simulink model "dspvorbisdec"  (Simulink 8.3)
settings: Solver=FixedStepDiscrete  SolverMode=SingleTasking  StartTime=0.0  StopTime=inf  RelTol=1e-3
PostLoadFcn:
  | hws  = get_param(bdroot,'modelworkspace');
  | dspvorbisdec_SampRt = hws.evalin('dspvorbisdec_OutputSampRt');
  | clear hws;
StopFcn:
  | dspvorbisdec_hws = get_param(bdroot,'modelworkspace');
  | dspvorbisdec_tmp = dspvorbisdec_hws.data;
  | for i = 1:length(dspvorbisdec_tmp)
  |   if strcmp(dspvorbisdec_tmp(i).Name,'dspvorbisdec_OutputSampRt')
  |      if (dspvorbisdec_tmp(i).Value~=dspvorbisdec_SampRt)
  |         dspvorbisdec_hws.assignin('dspvorbisdec_OutputSampRt', dspvorbisdec_SampRt);
  |      end
  |   end
  | end
  | 
  | clear hws dspvorbisdec_tmp i dspvorbisdec_hws;
undefined symbols (not defined in the file or in its folder): blockSize, errordlg, uiwait, warndlg
libraries: simulink x5, dspmtrx3 x3, dspindex x2, dspsigops x1, dspxfrm3 x1, dspmisc x1, dspsnks4 x1, dspsrcs4 x1
(part 2 of 3)

== matlab function Decode All Pages of Data/decodePage/Decode Audio/Decode an Audio Block/Decode Floor and Residue (4.3.2-4.3.5) ==
  data: resiOut output double; floor1Out output double; ifOutput output double; blockSize input uint32; startBitPoint input double; mapNum input double; dat input double; mapData input double; codeBooks input double; resiData input double; resiDataLocs input double; floor1Data input double; floor1DataLocs input double; numChannels input double; totalBytes input double
function [resiOut, floor1Out, ifOutput] = decodeFloorResidue(blockSize, startBitPoint, mapNum, dat, mapData, codeBooks, resiData, resiDataLocs, floor1Data, floor1DataLocs, numChannels, totalBytes)

persistent floor1_step2_flag1;
if isempty(floor1_step2_flag1)
    floor1_step2_flag1 = uint8(zeros(256,1));
end
persistent floor1_final_Y1;
if isempty(floor1_final_Y1)
    floor1_final_Y1 = uint32(zeros(256,1));
end
persistent floor1_step2_flag;
if isempty(floor1_step2_flag)
    floor1_step2_flag = uint8(zeros(256,1));
end
persistent floor1_final_Y;
if isempty(floor1_final_Y)
    floor1_final_Y = uint32(zeros(256,1));    
end
persistent classifications;
if isempty(classifications)
    classifications = uint32(zeros(256,2)); 
end
persistent uzeros8192;
if isempty (uzeros8192)
    uzeros8192 = uint8(zeros(8192,2));
end
persistent zeros8192;
if isempty(zeros8192)
    zeros8192 = double(zeros(8192,2));
end
persistent zeros256;
if isempty(zeros256)
    zeros256 = uint8(zeros(256,1));
end

persistent data;
if isempty(data)
    data = logical(false(16384, 1));
end
for m = uint32(0):uint32(totalBytes-1)
    for i = eml.unroll(uint32(1):uint32(8))
        data(8*m+i) = bitget(dat(m+1), i); % convert bytestream into bitstream
    end
end


%%%%%%%%%%%%%%%%%%%%%%%%%%%%%%%%%%%%%%%%%%%%%%%%%%%%%%%%%%%%%%%%%%%%%%%%
%%%%%%%%%%%% Decode Floor1 %%%%%%%%%%%%%%%%%%%%%%%%%%%%%%%%%%%%%%%%%%%%%
%%%%%%%%%%%%%%%%%%%%%%%%%%%%%%%%%%%%%%%%%%%%%%%%%%%%%%%%%%%%%%%%%%%%%%%%
% Decoding routines below follow Part 7.2.2 of Vorbis Decoder Specification, most names of variables and parameters are unchanged for better readibility 

bitPoint = startBitPoint;
floor1Out = uzeros8192; % enforce memcpy at code generation
resiOut = zeros8192; % enforce memcpy at code generation

no_residue = uint8(zeros(2,1));
curFloorLen = blockSize/2;

mapNum = mapNum*2;

%Iterate over each channel of 2 channels
for i_ch = 1:numChannels
    bytePoint = uint32(1);
    
    % Check if [no_residue] is set
    bitPoint = bitPoint + uint32(1);
    if ~data(bitPoint-1)
        no_residue(i_ch) = 1;
        continue;
    end
    
    submap_number = mapData(1+mapNum+2, i_ch);
    floor_number = mapData(1+mapNum+2, numChannels+submap_number*2+1)+1;
    
    a = uint32([256, 128, 86, 64]);
    range1 = a(floor1Data(floor1DataLocs(4,floor_number)));

    % ilog() function from the original C-library
    ret = uint32(0);
    v = uint32(range1-1);
    while (v)
        ret = ret+1;
        v = bitshift(v,-1);
    end
    % end of ilog()
    count = ret;

    floor1_Y = zeros256;
    for j = eml.unroll(uint32(1):uint32(2))
        for i = uint32(1):count
            floor1_Y(bytePoint) = bitset(floor1_Y(bytePoint), i, data(bitPoint)); 
            bitPoint = bitPoint + 1;
        end
        bytePoint = bytePoint + 1;
    end

    offset = uint32(2);
    for iter = 0:floor1Data(floor1DataLocs(1,floor_number))-1
        class1 = floor1Data(floor1DataLocs(2,floor_number)+iter);
        ix1 = class1+1+(floor_number-1)*16;
        cdim =  floor1Data(floor1DataLocs(3,ix1));
        cbits = floor1Data(floor1DataLocs(3,ix1)+1);
        csub = bitshift(uint32(1),cbits)-1;
        cval = uint32(0);
        if (cbits)
            book = floor1Data(floor1DataLocs(3,ix1)+2)+1;
            %HUFFMAN DECODE
            huff_bit_count = uint32(0);
            huff_buf = uint32(0);
            ifdecoded = false;
            while (~ifdecoded)
                huff_bit_count = huff_bit_count + 1;
                huff_buf = bitset(huff_buf, huff_bit_count, data(bitPoint));
                for iter_h = codeBooks(2*book-1, 256*30-32+huff_bit_count-1):(codeBooks(2*book-1, 256*30-32+huff_bit_count)-1)
                    if (huff_buf==bitand(codeBooks(2*book, iter_h), bitshift(uint32(1), huff_bit_count)-1))
                        if huff_bit_count == codeBooks(2*book-1, 2+iter_h)
                            cval = codeBooks(2*book, iter_h+codeBooks(2*book-1, 2))-1;
                            ifdecoded = true;
                        end
                        break;
                    end
                end
                bitPoint = bitPoint + 1;
            end
            %END HUFFMAN DECODE                
        end

        for iter_j = 0:cdim-1
            if (cbits)
                book = floor1Data(floor1DataLocs(3,ix1)+3+bitand(cval, csub))+1;
            else
                book = floor1Data(floor1DataLocs(3,ix1)+2+bitand(cval, csub))+1;
            end
            cval = uint32(bitshift(cval, -int32(cbits)));                                                    
            if (book~=256)
                %HUFFMAN DECODE
                huff_bit_count = uint32(0);
                huff_buf = uint32(0);
                ifdecoded = false;
                while (~ifdecoded)
                    huff_bit_count = huff_bit_count + 1;
                    huff_buf = bitset(huff_buf, huff_bit_count, data(bitPoint));
                    for iter_h = codeBooks(2*book-1, 256*30-32+huff_bit_count-1):(codeBooks(2*book-1, 256*30-32+huff_bit_count)-1)
                        if (huff_buf==bitand(codeBooks(2*book, iter_h), bitshift(uint32(1), huff_bit_count)-1))
                            if huff_bit_count == codeBooks(2*book-1, 2+iter_h)
                                floor1_Y(iter_j+offset+1) = codeBooks(2*book, iter_h+codeBooks(2*book-1, 2))-1;
                                ifdecoded = true;
                            end
                            break;                            
                        end
                    end
                    bitPoint = bitPoint + 1;
                end
                %END HUFFMAN DECODE                
            else
                floor1_Y(iter_j+offset+1) = 0;
            end
        end
        offset = offset + cdim;
    end

    % CURVE COMPUTATION
    floor1_step2_flag(1) = 1;
    floor1_step2_flag(2) = 1;                                
    floor1_final_Y(1) = floor1_Y(1);
    floor1_final_Y(2) = floor1_Y(2);
    
    flIx = floor1DataLocs(5, floor_number); % remember this index for further multiple use

    for m = uint32(2):floor1Data(floor1DataLocs(1, floor_number)-1)-1
        % low_neighbor, hi_neigbor
        low_neighbor_offset = uint32(0);
        hi_neighbor_offset = uint32(1);
        lx = int32(0); 
        hx = int32(curFloorLen);
        for q = uint32(0):(m-1)
            if (floor1Data(flIx+q)<floor1Data(flIx+m))
                if (floor1Data(flIx+q)>lx)
                    low_neighbor_offset = q; lx=int32(floor1Data(flIx+q));
                end
            end
            if (floor1Data(flIx+q)>floor1Data(flIx+m))
                if (floor1Data(flIx+q)<hx)
                    hi_neighbor_offset = q; hx=int32(floor1Data(flIx+q));
                end
            end
        end
        %%%%%%%%%%%%%% end %%%%%%%%%%%%%%%%%%

        x0 = int32(floor1Data(flIx+low_neighbor_offset));
        y0 = int32(floor1_final_Y(low_neighbor_offset+1));
        x1 = int32(floor1Data(flIx+hi_neighbor_offset));
        y1 = int32(floor1_final_Y(hi_neighbor_offset+1));
        X = int32(floor1Data(flIx+m));

        % render_point(x0, y0, x1, y1, X)
        dy = y1-y0;
        adx = x1-x0;
        ady = abs(dy);
        err = ady*(X-x0);
        if (adx==0); adx=int32(1); end
        off = (err-rem(err,adx))/adx;
        if (dy<0)
            predicted = y0 - off;
        else
            predicted = y0 + off;
        end
        %%%%%%% end %%%%%%%%%%%%%%

        val = int32(floor1_Y(m+1)); 
        highroom = int32(range1)-predicted;
        lowroom = predicted;
        if (highroom<lowroom)
            room = highroom*2;
        else
            room = lowroom*2;
        end
        if (val)
            floor1_step2_flag(low_neighbor_offset+1) = 1;
            floor1_step2_flag(hi_neighbor_offset+1) = 1;                                        
            floor1_step2_flag(m+1) = 1;
            if val>=room
                if highroom>lowroom
                    floor1_final_Y(m+1) = val-lowroom+predicted;
                else
                    floor1_final_Y(m+1) = predicted-val+highroom-1;
                end
            else
                if (mod(val, 2))
                    floor1_final_Y(m+1) = predicted-(val+1)/2;
                else
                    floor1_final_Y(m+1) = predicted+val/2;
                end
            end
        else
            floor1_step2_flag(m+1) = 0;
            floor1_final_Y(m+1) = predicted;
        end
    end

    n = floor1Data(floor1DataLocs(1, floor_number)-1);
    c = 333333*ones(256, 1);
    for m = flIx:(flIx+n-1)
        c(m-flIx+1) = floor1Data(m);
    end
    [floor1_X_list1, ix] = sort(c);
    for m = 1:n
        floor1_final_Y1(m) = floor1_final_Y(ix(m));
        floor1_step2_flag1(m) = floor1_step2_flag(ix(m));        
    end

    hx = int32(0);
    lx = int32(0);
    hy = int32(0);
    floor1_multiplier = floor1Data(floor1DataLocs(4,floor_number));
    ly = int32(floor1_final_Y1(1)*floor1_multiplier);
    for m = 1:(floor1Data(floor1DataLocs(1, floor_number)-1)-1)
        if (floor1_step2_flag1(m+1))
            hy = int32(floor1_final_Y1(m+1)*floor1_multiplier);
            hx = int32(floor1_X_list1(m+1));

            % Floor rendering routines
            dy = hy - ly;
            adx = hx-lx;
            ady = abs(dy);
            if (adx==0); adx=int32(1); end
            base = (dy-rem(dy,adx))/adx;
            x = lx;
            y = ly;
            err = int32(0);
            if (dy<0); sy = base - 1;
            else sy = base + 1; end
            ady = ady - abs(base)*adx;
            floor1Out(x+1,i_ch) = y;
            
            for x = lx+2:hx
                err = err + ady;
                if (err>=adx)
                    err = err - adx;
                    y = y + sy;
                else
                    y = y + base;
                end

                floor1Out(x,i_ch) = y;
            end            
            % end of line rendering
            lx = hx;
            ly = hy;
        end
    end

    if (hx<=int32(curFloorLen))
        % line rendering routines again
        dy = int32(0);
        adx = int32(curFloorLen) - hx;
        ady = abs(dy);
        if (adx==0); adx=int32(1); end
        base = (dy-rem(dy,adx))/adx;
        x = hx;
        y = hy;
        err = int32(0);
        if (dy<0)
            sy = base - 1;
        else
            sy = base + 1;
        end
        ady = ady - abs(base)*adx;
        floor1Out(x+1,i_ch) = y;
        for x = hx+2:int32(curFloorLen)
            err = err + ady;
            if (err>=adx)
                err = err - adx;
                y = y + sy;
            else
                y = y + base;
            end
            floor1Out(x,i_ch) = y;
        end
        % end of line rendering
    end

end

%%%%%%%%%%%%%%%%%%%%%%%%%%%%%%%%%%%%%%%%%%%%%%%%%%%%%%%%%%%%%%%%%%%%%%%%
%%%%%%%%%%%%%%%%%%%%% Decode residue %%%%%%%%%%%%%%%%%%%%%%%%%%%%%%%%%%%
%%%%%%%%%%%%%%%%%%%%%%%%%%%%%%%%%%%%%%%%%%%%%%%%%%%%%%%%%%%%%%%%%%%%%%%%
% Decoding routines below follow Part 8.6.2 of Vorbis Decoder Specification, most names of variables and parameters are unchanged for better readibility 

if (sum(no_residue)*(numChannels==1)+(sum(no_residue)-1)*(numChannels==2))>0
    ifOutput = 0; % no audio energy in the frame
else
    ifOutput = 1;
end

% 4.3.3 of Vorbis Decoder Specification, nonzero vector propagate
if (mapData(1+mapNum+1,2)>0) % To Avoid overflow error
    for i_sub = 0:mapData(1+mapNum+1,2)-1
        if (~no_residue(mapData(1+mapNum+1,3+i_sub*2)+1))||(~no_residue(mapData(1+mapNum+1,3+i_sub*2+1)+1))
            no_residue(mapData(1+mapNum+1,3+i_sub*2)+1) = 0;
            no_residue(mapData(1+mapNum+1,3+i_sub*2+1)+1) = 0;
        end
    end
end

vorbis_mapping_submaps = mapData(1+mapNum+1,1);
for i_sub = 1:vorbis_mapping_submaps % Iterate vorbis_mapping_submaps times
    do_not_decode_flag = uint8(zeros(2,1));
    ch_tmp = uint32(0);
    for j_ch = uint32(0):numChannels-1
        if (mapData(1+mapNum+2,j_ch+1)==i_sub-1)
            if (no_residue(j_ch+1))
                do_not_decode_flag(ch_tmp+1) = 1;
            end
            ch_tmp = ch_tmp + 1;
        end
    end

    resi_number = mapData(1+mapNum+2,numChannels+i_sub*2)+1; 
    resi_type = resiData(resiDataLocs(1,resi_number)-2);

    ch = ch_tmp;
    if (resi_type == 2)
        ch = uint32(1);
    end
    
    book = resiData(resiDataLocs(1,resi_number)+10)+1;
    classwords_per_codeword = int32(codeBooks(2*book-1, 1));

    residue_begin = resiData(resiDataLocs(1,resi_number))+bitshift(uint32(resiData(resiDataLocs(1,resi_number)+1)), 8)+bitshift(uint32(resiData(resiDataLocs(1,resi_number)+2)), 16);
    residue_end = resiData(resiDataLocs(1,resi_number)+3)+bitshift(uint32(resiData(resiDataLocs(1,resi_number)+4)), 8)+bitshift(uint32(resiData(resiDataLocs(1,resi_number)+5)), 16);
    residue_partition_size = resiData(resiDataLocs(1,resi_number)+6)+bitshift(uint32(resiData(resiDataLocs(1,resi_number)+7)), 8)+bitshift(uint32(resiData(resiDataLocs(1,resi_number)+8)), 16) + 1;
    n_to_read = residue_end - residue_begin;
    partitions_to_read = n_to_read/residue_partition_size;

    iter_step = 1;
    for iter_pass = uint32(0):resiData(resiDataLocs(1,resi_number)-1)-1 %look->stages loop
        partition_count = 0;
        while partition_count<partitions_to_read % partvals loop
            if (iter_pass==0)
                for j_ch = uint32(1):ch
                    if (do_not_decode_flag(j_ch)); continue; end;
                    
                    %HUFFMAN DECODE
                    huff_bit_count = uint32(0);
                    huff_buf = uint32(0);
                    temp = uint32(0);
                    ifdecoded = false;
                    while (~ifdecoded)
                        huff_bit_count = huff_bit_count + 1;
                        huff_buf = bitset(huff_buf, huff_bit_count, data(bitPoint));
                        for iter_h = codeBooks(2*book-1, 256*30-32+huff_bit_count-1):(codeBooks(2*book-1, 256*30-32+huff_bit_count)-1)
                            if (huff_buf==bitand(codeBooks(2*book, iter_h), bitshift(uint32(1), huff_bit_count)-1))
                                if huff_bit_count == codeBooks(2*book-1, 2+iter_h)
                                    temp = codeBooks(2*book, iter_h+codeBooks(2*book-1, 2))-1;
                                    ifdecoded = true;
                                end
                                break;
                            end
                        end
                        bitPoint = bitPoint + 1;
                    end
                    %END HUFFMAN DECODE                    
                    for k = (classwords_per_codeword-1):-1:0
                        classifications(k+partition_count+1,j_ch) = mod(temp, resiData(resiDataLocs(1,resi_number)+9)); % Modified for stereo
                        temp = (temp-classifications(k+partition_count+1,j_ch))/resiData(resiDataLocs(1,resi_number)+9);
                    end
                end
            end


            for iter_i = 0:(classwords_per_codeword-1)
                if (partition_count<partitions_to_read)
                    for j_ch = 1:ch
                        if (do_not_decode_flag(j_ch));
                            partition_count = partition_count + 1;                            
                            continue; 
                        end;                        
                        vqclass1 = classifications(partition_count+1,j_ch);% Modified for stereo
                        vqbook = resiData(resiDataLocs(2, resi_number)+vqclass1*8 + iter_pass) + 1;
                        vqIx = vqbook*2;
                        if (vqbook~=256)

                            offset = residue_begin+partition_count*residue_partition_size;
                            step = uint32(0);
                            switch resi_type
                                case 0
                                    step = (residue_partition_size-rem(residue_partition_size,codeBooks(vqIx-1, 1)))/codeBooks(vqIx-1, 1);
                                case {1, 2}
                                    step = residue_partition_size;
                            end

                            while (iter_step<=step)

                                %HUFFMAN DECODE
                                huff_bit_count = uint32(0);
                                huff_buf = uint32(0);
                                lookup_offset = uint32(0);
                                ifdecoded = false;
                                while (~ifdecoded)
                                    huff_bit_count = huff_bit_count + 1;
                                    huff_buf = uint32(bitset(huff_buf, huff_bit_count, data(bitPoint)));
                                    for iter_h = codeBooks(vqIx-1, 256*30-32+huff_bit_count-1):(codeBooks(vqIx-1, 256*30-32+huff_bit_count)-1)
                                        if (huff_buf==bitand(codeBooks(vqIx, iter_h), bitshift(uint32(1), huff_bit_count)-1))
                                            if huff_bit_count == codeBooks(vqIx-1, 2+iter_h)
                                                lookup_offset = codeBooks(vqIx, iter_h+codeBooks(vqIx-1, 2))-1;
                                                ifdecoded = true;
                                            end
                                            break;
                                        end
                                    end
                                    bitPoint = bitPoint + 1;
                                end
                                %END HUFFMAN DECODE                    


                                xr = codeBooks(vqIx-1, 3+codeBooks(vqIx-1, 2)+1);
                                mantissa = double(bitand(xr, 2097151));
                                sign1 = bitand(xr, 2147483648);
                                exponent = double(bitshift(uint32(bitand(xr, 2145386496)), -21));
                                if sign1; mantissa=-mantissa; end
                                codebook_minimum_value = int32(mantissa*(2^(exponent-788)));                        

                                xr = codeBooks(vqIx-1, 3+codeBooks(vqIx-1, 2)+2);
                                mantissa = double(bitand(xr, 2097151));
                                sign1 = bitand(xr, 2147483648);
                                exponent = double(bitshift(uint32(bitand(xr, 2145386496)), -21));
                                if sign1; mantissa=-mantissa; end
                                codebook_delta_value = int32(mantissa*(2^(exponent-788))); 
                                value_vector = int32(zeros(32,2)); 

                                if (codeBooks(vqIx-1, 3+codeBooks(vqIx-1, 2))==1)
                                    last = int32(0);
                                    index_divisor = uint32(1);
                                    for iter_h = 0:(codeBooks(vqIx-1, 1)-1)
                                        multiplicand_offset = mod((lookup_offset-mod(lookup_offset,index_divisor))/index_divisor, codeBooks(vqIx-1, 3+codeBooks(vqIx-1, 2)+5));
                                        value_vector(iter_h+1, j_ch) = int32(codeBooks(vqIx-1, 3+codeBooks(vqIx-1, 2)+6+multiplicand_offset))*codebook_delta_value+codebook_minimum_value+last;
                                        if (codeBooks(vqIx-1, 3+codeBooks(vqIx-1, 2)+4))
                                            last = value_vector(iter_h+1, j_ch);
                                        end
                                        index_divisor = index_divisor*codeBooks(vqIx-1, 3+codeBooks(vqIx-1, 2)+5);
                                    end
                                else
                                   last = int32(0);
                                   multiplicand_offset = lookup_offset*codeBooks(vqIx-1, 1);
                                   for iter_h = 0:(codeBooks(vqIx-1, 1)-1)
                                       value_vector(iter_h+1, j_ch) = int32(codeBooks(vqIx-1, 3+codeBooks(vqIx-1, 2)+6+multiplicand_offset))*codebook_delta_value+codebook_minimum_value+last;
                                       if (codeBooks(vqIx-1, 3+codeBooks(vqIx-1, 2)+4))
                                           last = value_vector(iter_h+1, j_ch);
                                       end
                                       multiplicand_offset = multiplicand_offset + 1;
                                   end
                               end

                               switch resi_type
                                   case 0
                                       for iter_h = 0:(codeBooks(vqIx-1, 1)-1)
                                           resiOut(offset+1+iter_step+iter_h*step, j_ch) = resiOut(offset+1+iter_step+iter_h*step, j_ch)+double(value_vector(iter_h+1, j_ch)); % modified for stereo
                                       end
                                   case {1,2}
                                       for iter_h = 0:(codeBooks(vqIx-1, 1)-1)
                                           resiOut(offset+iter_step, j_ch) = resiOut(offset+iter_step, j_ch)+double(value_vector(iter_h+1, j_ch)); % modified for stereo
                                           iter_step = iter_step + 1;                                            
                                       end
                                end
                           end
                           iter_step = 1;
                       end
                       partition_count = partition_count + 1;
                    end
               end
           end
       end
    end

% Post-decoding step for resi_type == 2
    if (resi_type==2)
        for i = uint32(1):curFloorLen
            for j = eml.unroll(uint32(1):uint32(2))
                if j>ch_tmp; break; end;
                resiOut(i,j) = resiOut((i-1)*ch_tmp + j,1);
            end
        end
    end

    ch = uint32(0);
    resiTmp = resiOut;
    for j_ch = uint32(0):numChannels-1
        if (mapData(1+mapNum+2,j_ch+1)==i_sub-1)
            resiOut(:,j_ch+1) = resiTmp(:,ch+1);
            ch = ch + 1;
        end
   end
    
end


%% Inverse Coupling, Part 4.3.5
for i_coup = int32(mapData(1+mapNum+1,2))-1:-1:int32(0)
     mag_ix = mapData(1+mapNum+1,3+i_coup*2)+1;
     angle_ix = mapData(1+mapNum+1,3+i_coup*2+1)+1;
     for i = uint32(1):curFloorLen 
         if resiOut(i,mag_ix)>0
             if resiOut(i,angle_ix)>0
                 new_M = resiOut(i,mag_ix);
                 new_A = resiOut(i,mag_ix) - resiOut(i,angle_ix);
             else
                 new_A = resiOut(i,mag_ix);
                 new_M = resiOut(i,mag_ix) + resiOut(i,angle_ix);
             end
         else
             if resiOut(i,angle_ix)>0
                 new_M = resiOut(i,mag_ix);
                 new_A = resiOut(i,mag_ix) + resiOut(i,angle_ix);
             else
                 new_A = resiOut(i,mag_ix);
                 new_M = resiOut(i,mag_ix) - resiOut(i,angle_ix);
             end             
         end
         resiOut(i,mag_ix) = new_M;
         resiOut(i,angle_ix) = new_A;
     end
end

if (numChannels==1) % fix to have sound from both speakers even in mono mode
    floor1Out(:,2) = floor1Out(:,1);
    resiOut(:,2) = resiOut(:,1);
end

== stateflow chart Decode All Pages of Data ==
  state [decodedPage,decodedPageSize,adjCount] = decodePage(dataPage,pageCount,segmentTable,numSegments,numBytes,ifUnpack) [function]
  state Decoding/ [parallel]
    settings: executionOrder=1
    state CountDown22Bytes/
      du:count=count+1;
    state BufferWholePage/
      du:dataPage[count]=b;count=count+1;
    state ReadSegmentationTable/
      en:nSeg=b;segTable=zeroTable;
      du:segTable[count]=b;count=count+1;
      nBytes=nBytes+uint16(b);
    state SyncToBeginning
      state CatchSymbol_O
      state CatchSymbol_g
      state CatchSymbol_g_again
      state CatchSymbol_S
      CatchSymbol_g_again -> CatchSymbol_O [order 2]
      CatchSymbol_g -> CatchSymbol_O [order 2]
      CatchSymbol_S -> CatchSymbol_O [order 2]
      CatchSymbol_O -> CatchSymbol_g : [b==79]
      (default) -> CatchSymbol_g
      CatchSymbol_g -> CatchSymbol_g_again [order 1] : [b==103]
      CatchSymbol_g_again -> CatchSymbol_S [order 1] : [b==103]
    (default) -> SyncToBeginning
    (junction 53) -> (junction 52) [order 1] : [decodedPageSize>0]{pageComplete;}
    (junction 53) -> (junction 52) [order 2]
    CountDown22Bytes -> ReadSegmentationTable : [count==23]{count=0;nBytes=0;}
    ReadSegmentationTable -> BufferWholePage : [count==nSeg]{count=1;dataPage[0]=b;}
    BufferWholePage -> (junction 53) : [count==nBytes]{[numRem]=processTable();
        | [decodedPage,decodedPageSize,pCount] = decodePage(dataPage,pCount,segTable,nSeg,nBytes,ifUnpack);}
    (junction 52) -> CatchSymbol_g [order 2]
    (junction 52) -> CatchSymbol_O [order 1] : [b~=79]
    CatchSymbol_S -> CountDown22Bytes [order 1] : [b==83]{count=1;pCount=pCount+1;}
  state ResetPageCounter/ [parallel]
    settings: executionOrder=2
    state CatchNumber_1
    state CatchSymbol_V
    state ResetCounter
    state CatchSymbol_s
    state CatchSymbol_i
    state CatchSymbol_b
    state CatchSymbol_r
    state CatchSymbol_o
    (default) -> CatchNumber_1
    CatchSymbol_V -> CatchNumber_1 [order 2]
    CatchSymbol_b -> CatchNumber_1 [order 2]
    ResetCounter -> CatchNumber_1
    CatchSymbol_s -> CatchNumber_1 [order 2]
    CatchSymbol_r -> CatchNumber_1 [order 2]
    CatchSymbol_o -> CatchNumber_1 [order 2]
    CatchSymbol_i -> CatchNumber_1 [order 2]
    CatchNumber_1 -> CatchSymbol_V : [b==1]
    CatchSymbol_V -> CatchSymbol_o [order 1] : [b==118]
    CatchSymbol_o -> CatchSymbol_r [order 1] : [b==111]
    CatchSymbol_r -> CatchSymbol_b [order 1] : [b==114]
    CatchSymbol_b -> CatchSymbol_i [order 1] : [b==98]
    CatchSymbol_i -> CatchSymbol_s [order 1] : [b==105]
    CatchSymbol_s -> ResetCounter [order 1] : [b==115]{pCount=1;
        | ifUnpack=false;
        | numRem=0;}
  data: dataPage function_input uint8 size=5500; pageCount function_input uint16 size=1; segmentTable function_input uint16 size=255; numSegments function_input uint16 size=1; numBytes function_input uint16 size=1; ifUnpack function_input boolean size=1; decodedPage function_output double; decodedPageSize function_output double; adjCount function_output double; newNumRem function_output double; decodedPage output double size=[55000 2]; count local uint16; decodedPageSize output int32; pCount local uint16 =uint16(0); segTable local uint16 size=255; nSeg local uint8; b input double; dataPage local uint8 size=5500; nBytes local uint16 =uint16(0); zeroTable local uint8 size=255 =uint8(zeros(255,1)); remData local uint8 size=765; ifUnpack local boolean size=1; numRem local double =0
  events: pageComplete output FUNCTION_CALL_EVENT
  function newNumRem  = processTable:
    | function newNumRem  = processTable
    | % These routines process the segmentation table of the current page and take care of 
    | % the problem of logical packets that span two consecutive pages
    | % Please refer to http://xiph.org/vorbis/doc/framing.html for details about Ogg Format
    | 
    | persistent zeros255 newRemData newSegTable;
    | if isempty(zeros255) 
    |     zeros255    = zeros(255,1,'uint16'); 
    |     newRemData  = zeros(765,1,'uint8'); 
    |     newSegTable = zeros255; 
    | end 
    | 
    | newNumRem = 0;
    | 
    | if (segTable(nSeg)==255) % See if there is a trailing segment in the current page that spans the current and the next pages
    |     if (pCount>2)
    |         while (segTable(nSeg)==255)
    |             newNumRem = newNumRem + 1;
    |             segTable(nSeg)=0;
    |             nSeg = nSeg-1;
    |         end
    |         for j = 1:newNumRem
    |             % Keep a trailing incomplete logical packet to concatenate with the next page
    |             newRemData(255*(j-1)*ones(255,1)+[1:255]') = dataPage((double(nBytes)-j*255)*ones(255,1)+[1:255]'); 
    |         end
    |         nBytes = nBytes-newNumRem*255;            
    |     end
    | elseif (pCount==2)
    |     ifUnpack = true;
    | end
    | 
    | % Concatenate the current page with an incomplete logical packet (if any) from the previous page.
    | for j = 1:numRem    
    |     segTable = [255;segTable(1:254)];
    |     nSeg = nSeg+1;
    |     dataPage = [remData(255*(j-1)*ones(255,1)+[1:255]'); dataPage(1:(5500-255))];
    |     nBytes = nBytes + 255;
    | end
    | 
    | % Convert the table into format that marks beginning of every logical packet in the current page
    | c = 1;
    | newSegTable = zeros255;
    | for i = 1:(nSeg-1)
    |     newSegTable(c) = newSegTable(c)+segTable(i);
    |     if (segTable(i)~=255)
    |         c = c+1;
    |         if (c~=1)
    |             newSegTable(c) = newSegTable(c)+newSegTable(c-1);
    |         end
    |     end
    | end
    | newSegTable(c) = newSegTable(c)+segTable(nSeg);
    | nSeg = uint8(c);
    | 
    | remData = newRemData;
    | segTable = newSegTable;
